simulink model "NARMAX_SIM"  (R2015b)
settings: Solver=VariableStepAuto  StartTime=0  StopTime=20000  MaxStep=1  RelTol=1e-3
undefined symbols (not defined in the file or in its folder): Ts
libraries: slident x1
settings Model: Creator=gmiglio  LastModifiedBy=gmiglio

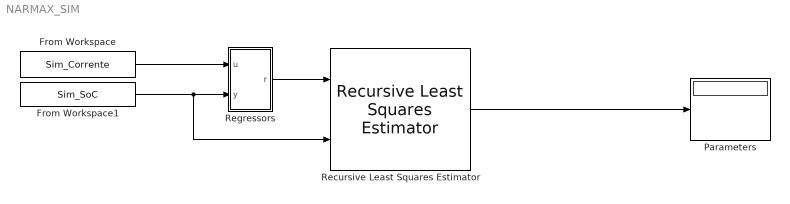
== system NARMAX_SIM ==
  From Workspace : FromWorkspace  VariableName=Sim_Corrente  SampleTime=0
  From Workspace1 : FromWorkspace  VariableName=Sim_SoC  SampleTime=0
  Parameters : Display
  Recursive Least Squares Estimator : slident/Estimators/Recursive Least Squares Estimator  InitialEstimateSource=None  InitialParameterData=3  P0=1e4  EstimationMethod=Forgetting Factor  AdaptationParameter=1  NormalizationBias=eps  OutputError=off  OutputP=off  AddEnablePort=off  Ts=Ts
  Regressors : Subsystem
  wires:
  Regressors/1(r) -> Recursive Least Squares Estimator/1
  From Workspace/1 -> Regressors/1(u)
  From Workspace1/1 -> Recursive Least Squares Estimator/2, Regressors/2(y)
  Recursive Least Squares Estimator/1 -> Parameters/1

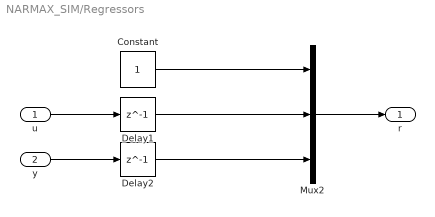
== system NARMAX_SIM/Regressors ==
  u : Inport
  y : Inport  Port=2
  Constant : Constant  SampleTime=Ts
  Delay1 : Delay  DelayLength=1  InitialCondition=0  SampleTime=Ts
  Delay2 : Delay  DelayLength=1  InitialCondition=0  SampleTime=Ts
  Mux2 : Mux  Inputs=3
  r : Outport
  wires:
  u/1 -> Delay1/1
  Mux2/1 -> r/1
  y/1 -> Delay2/1
  Delay2/1 -> Mux2/3
  Delay1/1 -> Mux2/2
  Constant/1 -> Mux2/1
